simulink model "simple_simulink_example"  (R2021a)
settings: Solver=FixedStepAuto  StartTime=0.0  StopTime=20  FixedStep=0.01  RelTol=1e-3
libraries: simulink x1
settings Model: Creator=Marcin  LastModifiedBy=Marcin

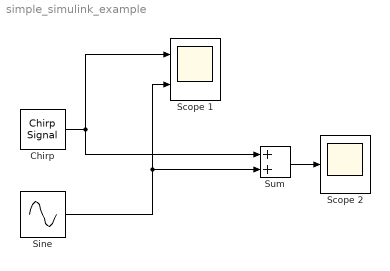
== system simple_simulink_example ==
  Chirp : simulink/Sources/Chirp Signal  f1=0.04  T=10  f2=1
  Scope 1 : Scope  NumInputPorts=2
  Scope 2 : Scope
  Sine : Sin  Amplitude=2  SampleTime=0
  Sum : Sum
  wires:
  Chirp/1 -> Scope 1/1, Sum/1
  Sine/1 -> Sum/2, Scope 1/2
  Sum/1 -> Scope 2/1
